simulink model "SmithVSPI"  (R2024b)
settings: Solver=VariableStepAuto  StartTime=0.0  StopTime=50000  FixedStep=10  RelTol=1e-3
undefined symbols (not defined in the file): n, p1, p2, p3, Vi
libraries: slpidlib x2
settings Model: Creator=HP  LastModifiedBy=HP

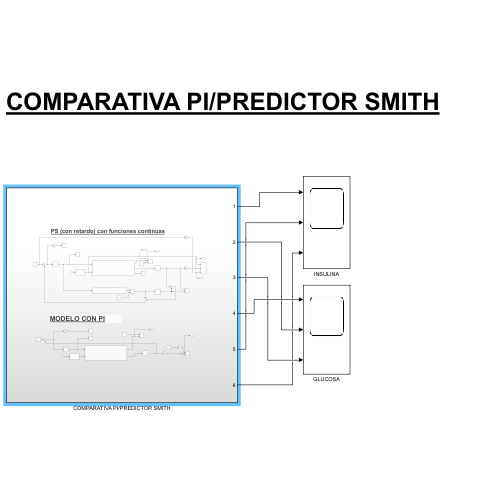
[thumbnail: Simulink's stored preview of the top-level diagram]
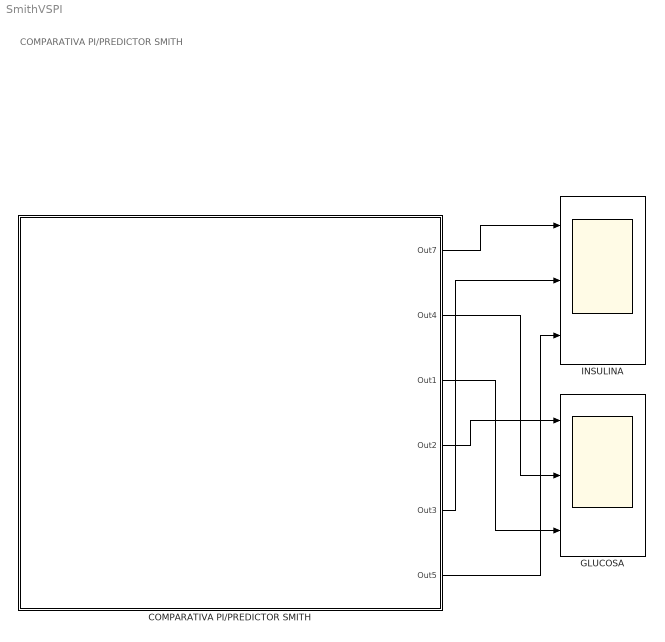
== system SmithVSPI ==
  note: COMPARATIVA PI/PREDICTOR SMITH
  COMPARATIVA PI/PREDICTOR SMITH : Subsystem
  GLUCOSA : Scope  NumInputPorts=3
  INSULINA : Scope  NumInputPorts=3
  wires:
  COMPARATIVA PI/PREDICTOR SMITH/2(Out4) -> GLUCOSA/2
  COMPARATIVA PI/PREDICTOR SMITH/3(Out1) -> GLUCOSA/3
  COMPARATIVA PI/PREDICTOR SMITH/4(Out2) -> GLUCOSA/1
  COMPARATIVA PI/PREDICTOR SMITH/1(Out7) -> INSULINA/1
  COMPARATIVA PI/PREDICTOR SMITH/5(Out3) -> INSULINA/2
  COMPARATIVA PI/PREDICTOR SMITH/6(Out5) -> INSULINA/3

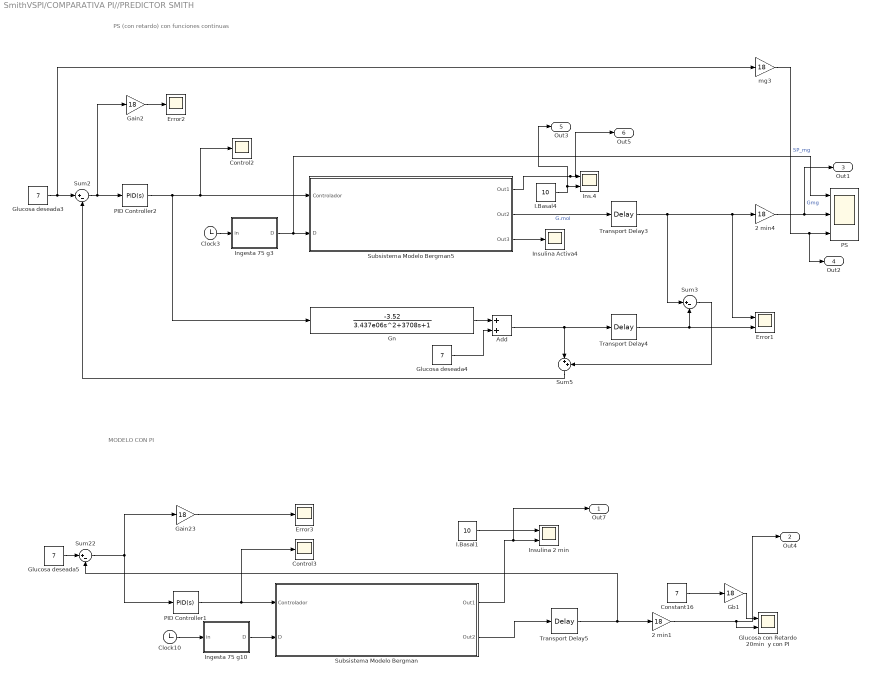
== system SmithVSPI/COMPARATIVA PI//PREDICTOR SMITH ==
  note: MODELO CON PI
  note: PS (con retardo) con funciones continuas
  2 min1 : Gain  Gain=18
  2 min4 : Gain  Gain=18
  Add : Sum
  Clock10 : Clock
  Clock3 : Clock
  Constant16 : Constant  Value=7
  Control2 : Scope
  Control3 : Scope
  Error1 : Scope  NumInputPorts=2
  Error2 : Scope
  Error3 : Scope
  Gain2 : Gain  Gain=18
  Gain23 : Gain  Gain=18
  Gb1 : Gain  Gain=18
  Glucosa con Retardo 20min  y con PI : Scope  NumInputPorts=2
  Glucosa deseada3 : Constant  Value=7
  Glucosa deseada4 : Constant  Value=7
  Glucosa deseada5 : Constant  Value=7
  Gn : TransferFcn  Numerator=[-3.52]  Denominator=[3.437e06 3708 1]
  I.Basal1 : Constant  Value=10
  I.Basal4 : Constant  Value=10
  Ingesta 75 g10 : MATLAB Function  TreatAsAtomicUnit=on
  Ingesta 75 g3 : MATLAB Function  TreatAsAtomicUnit=on
  Ins.4 : Scope  NumInputPorts=2
  Insulina 2 min : Scope  NumInputPorts=2
  Insulina Activa4 : Scope
  PID Controller1 : slpidlib/PID Controller  Controller=PID  Form=Parallel  TimeDomain=Continuous-time  UseExternalTs=off  SampleTime=-1  IntegratorMethod=Forward Euler  FilterMethod=Forward Euler  ControllerParametersSource=internal  P=-0.3195*1.5  I=-0.3195/2998.95  UseKiTs=off  D=0  UseExternalDerivativeSource=off  N=10  UseFilter=on  TunerSelectOption=Transfer Function Based (PID Tuner App)  InitialConditionSource=internal  InitialConditionForIntegrator=0  InitialConditionForFilter=0  DifferentiatorICPrevScaledInput=0  ExternalReset=none  TrackingMode=off  Kt=1  LimitOutput=on  SatLimitsSource=internal  UpperSaturationLimit=5  LowerSaturationLimit=0  LinearizeAsGain=on  AntiWindupMode=none  Kb=1  LimitIntegrator=off  UpperIntegratorSaturationLimit=inf  LowerIntegratorSaturationLimit=-inf  POutMin=[]  POutMax=[]  IOutMin=[]  IOutMax=[]  DOutMin=[]  DOutMax=[]  NOutMin=[]  NOutMax=[]  SumOutMin=[]  SumOutMax=[]  SaturationOutMin=[]  SaturationOutMax=[]  PParamMin=[]  PParamMax=[]  IParamMin=[]  IParamMax=[]  DParamMin=[]  DParamMax=[]  NParamMin=[]  NParamMax=[]  KbParamMin=[]  KbParamMax=[]  KtParamMin=[]  KtParamMax=[]  KbOutMin=[]  KbOutMax=[]  KtOutMin=[]  KtOutMax=[]  IntegratorOutMin=[]  IntegratorOutMax=[]  FilterOutMin=[]  FilterOutMax=[]  SumI1OutMin=[]  SumI1OutMax=[]  SumI2OutMin=[]  SumI2OutMax=[]  SumI3OutMin=[]  SumI3OutMax=[]  SumI4OutMin=[]  SumI4OutMax=[]  SumDOutMin=[]  SumDOutMax=[]  DifferentiatorOutMin=[]  DifferentiatorOutMax=[]  FilterDiffOutCoefMin=[]  FilterDiffOutCoefMax=[]  ReciprocalOutMin=[]  ReciprocalOutMax=[]  SumDenOutMin=[]  SumDenOutMax=[]  SumNumOutMin=[]  SumNumOutMax=[]  DivideOutMin=[]  DivideOutMax=[]  UdiffTsProdOutMin=[]  UdiffTsProdOutMax=[]  NTsProdOutMin=[]  NTsProdOutMax=[]  UintegralTsProdOutMin=[]  UintegralTsProdOutMax=[]  UngainTsProdOutMin=[]  UngainTsProdOutMax=[]  ClampingZeroOutDataTypeStr=Inherit: Inherit via back propagation  ClampingZeroOutMin=[]  ClampingZeroOutMax=[]  FilterDenConstantOutDataTypeStr=Inherit: Inherit via back propagation  FilterDenConstantOutMin=[]  FilterDenConstantOutMax=[]  PCopyOutDataTypeStr=Inherit: Inherit via back propagation  PCopyOutMin=[]  PCopyOutMax=[]  NCopyOutDataTypeStr=Inherit: Inherit via back propagation  NCopyOutMin=[]  NCopyOutMax=[]  IntegratorContinuousStateAttributes=''  IntegratorStateMustResolveToSignalObject=off  IntegratorRTWStateStorageClass=Auto  FilterContinuousStateAttributes=''  FilterStateMustResolveToSignalObject=off  FilterRTWStateStorageClass=Auto  ParallelPVariant=InternalParameters  IdealPVariant=Disabled  IVariant=InternalParameters  DVariant=InternalParameters  IntegratorVariant=Continuous  SatVariant=Enabled  AWVariant=Passthrough  PCopyVariant=Disabled  TRVariant=Disabled  FdbkBlocksVariant=Forward  IdealPFdbkVariant=Disabled  SatFdbkVariant=Disabled  DerivativeFilterVariant=ContFilter  NVariant=InternalParameters  NCopyVariant=Disabled  FilterICVariant=InternalICsFilter  IntegratorICVariant=InternalICs  ExternalResetVariant=Disabled  TRSumVariant=Passthrough  SumFdbkVariant=Disabled  SumVariant=Sum_PID  TsampFilterVariant=InternalTs  TsampNgainVariant=Passthrough  TsampIntegralVariant=Disabled_SignalSpec  ExternalSaturationOutDataTypeStr=Inherit: Same as second input  DerivativeSourceVariant=ErrorSignal  PreIntVariant=InternalPreInt
  PID Controller2 : slpidlib/PID Controller  Controller=PID  Form=Parallel  TimeDomain=Continuous-time  UseExternalTs=off  SampleTime=-1  IntegratorMethod=Forward Euler  FilterMethod=Forward Euler  ControllerParametersSource=internal  P=-0.3195*1.5  I=-0.3195/2998.95  UseKiTs=off  D=0  UseExternalDerivativeSource=off  N=10  UseFilter=on  TunerSelectOption=Transfer Function Based (PID Tuner App)  InitialConditionSource=internal  InitialConditionForIntegrator=0  InitialConditionForFilter=0  DifferentiatorICPrevScaledInput=0  ExternalReset=none  TrackingMode=off  Kt=1  LimitOutput=on  SatLimitsSource=internal  UpperSaturationLimit=5  LowerSaturationLimit=0  LinearizeAsGain=on  AntiWindupMode=none  Kb=1  LimitIntegrator=off  UpperIntegratorSaturationLimit=inf  LowerIntegratorSaturationLimit=-inf  POutMin=[]  POutMax=[]  IOutMin=[]  IOutMax=[]  DOutMin=[]  DOutMax=[]  NOutMin=[]  NOutMax=[]  SumOutMin=[]  SumOutMax=[]  SaturationOutMin=[]  SaturationOutMax=[]  PParamMin=[]  PParamMax=[]  IParamMin=[]  IParamMax=[]  DParamMin=[]  DParamMax=[]  NParamMin=[]  NParamMax=[]  KbParamMin=[]  KbParamMax=[]  KtParamMin=[]  KtParamMax=[]  KbOutMin=[]  KbOutMax=[]  KtOutMin=[]  KtOutMax=[]  IntegratorOutMin=[]  IntegratorOutMax=[]  FilterOutMin=[]  FilterOutMax=[]  SumI1OutMin=[]  SumI1OutMax=[]  SumI2OutMin=[]  SumI2OutMax=[]  SumI3OutMin=[]  SumI3OutMax=[]  SumI4OutMin=[]  SumI4OutMax=[]  SumDOutMin=[]  SumDOutMax=[]  DifferentiatorOutMin=[]  DifferentiatorOutMax=[]  FilterDiffOutCoefMin=[]  FilterDiffOutCoefMax=[]  ReciprocalOutMin=[]  ReciprocalOutMax=[]  SumDenOutMin=[]  SumDenOutMax=[]  SumNumOutMin=[]  SumNumOutMax=[]  DivideOutMin=[]  DivideOutMax=[]  UdiffTsProdOutMin=[]  UdiffTsProdOutMax=[]  NTsProdOutMin=[]  NTsProdOutMax=[]  UintegralTsProdOutMin=[]  UintegralTsProdOutMax=[]  UngainTsProdOutMin=[]  UngainTsProdOutMax=[]  ClampingZeroOutDataTypeStr=Inherit: Inherit via back propagation  ClampingZeroOutMin=[]  ClampingZeroOutMax=[]  FilterDenConstantOutDataTypeStr=Inherit: Inherit via back propagation  FilterDenConstantOutMin=[]  FilterDenConstantOutMax=[]  PCopyOutDataTypeStr=Inherit: Inherit via back propagation  PCopyOutMin=[]  PCopyOutMax=[]  NCopyOutDataTypeStr=Inherit: Inherit via back propagation  NCopyOutMin=[]  NCopyOutMax=[]  IntegratorContinuousStateAttributes=''  IntegratorStateMustResolveToSignalObject=off  IntegratorRTWStateStorageClass=Auto  FilterContinuousStateAttributes=''  FilterStateMustResolveToSignalObject=off  FilterRTWStateStorageClass=Auto  ParallelPVariant=InternalParameters  IdealPVariant=Disabled  IVariant=InternalParameters  DVariant=InternalParameters  IntegratorVariant=Continuous  SatVariant=Enabled  AWVariant=Passthrough  PCopyVariant=Disabled  TRVariant=Disabled  FdbkBlocksVariant=Forward  IdealPFdbkVariant=Disabled  SatFdbkVariant=Disabled  DerivativeFilterVariant=ContFilter  NVariant=InternalParameters  NCopyVariant=Disabled  FilterICVariant=InternalICsFilter  IntegratorICVariant=InternalICs  ExternalResetVariant=Disabled  TRSumVariant=Passthrough  SumFdbkVariant=Disabled  SumVariant=Sum_PID  TsampFilterVariant=InternalTs  TsampNgainVariant=Passthrough  TsampIntegralVariant=Disabled_SignalSpec  ExternalSaturationOutDataTypeStr=Inherit: Same as second input  DerivativeSourceVariant=ErrorSignal  PreIntVariant=InternalPreInt
  PS : Scope  NumInputPorts=3
  Subsistema Modelo Bergman : Subsystem
  Subsistema Modelo Bergman5 : Subsystem
  Sum2 : Sum  Inputs=|+-
  Sum22 : Sum  Inputs=|+-
  Sum3 : Sum  Inputs=|+-
  Sum5 : Sum  Inputs=|++
  Transport Delay3 : TransportDelay  DelayTime=900  InitialOutput=7
  Transport Delay4 : TransportDelay  DelayTime=900  InitialOutput=7
  Transport Delay5 : TransportDelay  DelayTime=1200  InitialOutput=7
  mg3 : Gain  Gain=18
  Out7 : Outport
  Out4 : Outport  Port=2
  Out1 : Outport  Port=3
  Out2 : Outport  Port=4
  Out3 : Outport  Port=5
  Out5 : Outport  Port=6
  wires:
  PID Controller1/1 -> Control3/1, Subsistema Modelo Bergman/1(Controlador)
  Subsistema Modelo Bergman/1(Out1) -> Out7/1, Insulina 2 min/2
  Glucosa deseada5/1 -> Sum22/1
  Subsistema Modelo Bergman/2(Out2) -> Transport Delay5/1
  Sum22/1 -> PID Controller1/1, Gain23/1
  Transport Delay5/1 -> Sum22/2, 2 min1/1
  Gb1/1 -> Glucosa con Retardo 20min  y con PI/1
  Ingesta 75 g10/1(D) -> Subsistema Modelo Bergman/2(D)
  I.Basal1/1 -> Insulina 2 min/1
  Gain23/1 -> Error3/1
  Clock10/1 -> Ingesta 75 g10/1(in)
  2 min1/1 -> Out4/1, Glucosa con Retardo 20min  y con PI/2
  Constant16/1 -> Gb1/1
  2 min4/1 -> Out1/1, PS/2  "Gmg"
  Add/1 -> Transport Delay4/1, Sum5/1
  Sum3/1 -> Sum5/2
  I.Basal4/1 -> Out3/1, Ins.4/2
  Gain2/1 -> Error2/1
  PID Controller2/1 -> Gn/1, Control2/1, Subsistema Modelo Bergman5/1(Controlador)
  Subsistema Modelo Bergman5/2(Out2) -> Transport Delay3/1  "G.mol"
  Subsistema Modelo Bergman5/3(Out3) -> Insulina Activa4/1
  Ingesta 75 g3/1(D) -> PS/1, Subsistema Modelo Bergman5/2(D)
  Gn/1 -> Add/1
  Subsistema Modelo Bergman5/1(Out1) -> Out5/1, Ins.4/1
  Sum5/1 -> Sum2/2
  Glucosa deseada4/1 -> Add/2
  mg3/1 -> Out2/1, PS/3  "SP_mg"
  Glucosa deseada3/1 -> mg3/1, Sum2/1
  Transport Delay3/1 -> Sum3/1, Error1/1, 2 min4/1
  Sum2/1 -> Gain2/1, PID Controller2/1
  Clock3/1 -> Ingesta 75 g3/1(in)
  Transport Delay4/1 -> Sum3/2, Error1/2

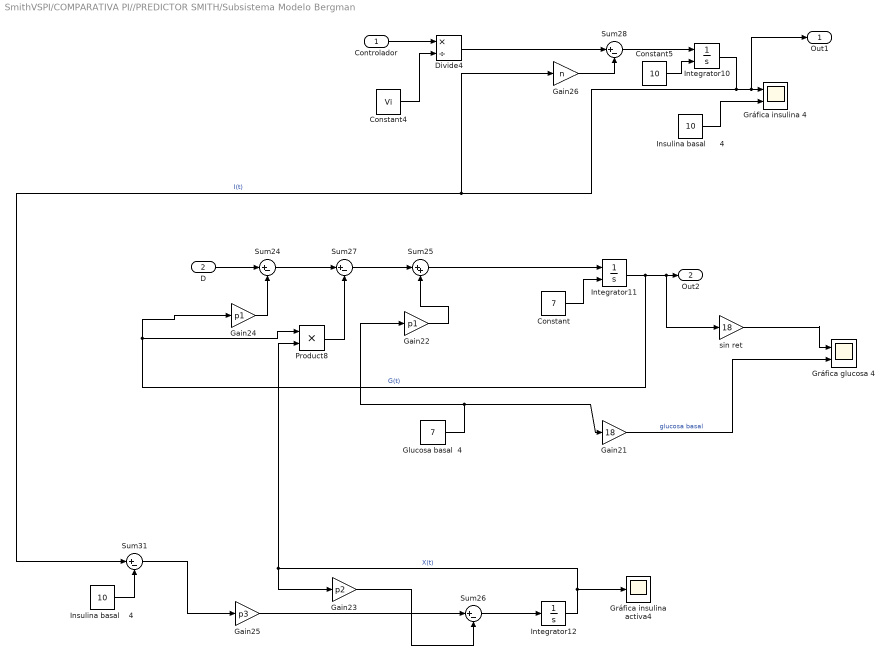
== system SmithVSPI/COMPARATIVA PI//PREDICTOR SMITH/Subsistema Modelo Bergman ==
  Controlador : Inport
  D : Inport  Port=2
  Constant : Constant  Value=7
  Constant4 : Constant  Value=Vi
  Constant5 : Constant  Value=10
  Divide4 : Product  Inputs=*/
  Gain21 : Gain  Gain=18
  Gain22 : Gain  Gain=p1
  Gain23 : Gain  Gain=p2
  Gain24 : Gain  Gain=p1
  Gain25 : Gain  Gain=p3
  Gain26 : Gain  Gain=n
  Glucosa basal  4 : Constant  Value=7
  Gráfica glucosa 4 : Scope  NumInputPorts=2
  Gráfica insulina 4 : Scope  NumInputPorts=2
  Gráfica insulina activa4 : Scope
  Insulina basal      4 : Constant  Value=10
  Insulina basal    4 : Constant  Value=10
  Integrator10 : Integrator  InitialConditionSource=external
  Integrator11 : Integrator  InitialConditionSource=external  InitialCondition=7
  Integrator12 : Integrator
  Product8 : Product
  Sum{24,26..28,31} (5 alike) : Sum  Inputs=|+-
  Sum25 : Sum  Inputs=|++
  sin ret : Gain  Gain=18
  Out1 : Outport
  Out2 : Outport  Port=2
  wires:
  Gain26/1 -> Sum28/2
  Glucosa basal  4/1 -> Gain22/1, Gain21/1
  D/1 -> Sum24/1
  Gain21/1 -> Gráfica glucosa 4/2  "glucosa basal"
  Integrator11/1 -> sin ret/1, Out2/1, Gain24/1, Product8/1  "G(t)"
  Integrator12/1 -> Product8/2, Gain23/1, Gráfica insulina activa4/1  "X(t)"
  Gain25/1 -> Sum26/1
  Integrator10/1 -> Out1/1, Gráfica insulina 4/1, Sum31/1, Gain26/1  "I(t)"
  Constant5/1 -> Integrator10/2
  Sum31/1 -> Gain25/1
  Sum26/1 -> Integrator12/1
  Gain23/1 -> Sum26/2
  Sum28/1 -> Integrator10/1
  Sum24/1 -> Sum27/1
  Sum25/1 -> Integrator11/1
  Gain24/1 -> Sum24/2
  Insulina basal      4/1 -> Gráfica insulina 4/2
  Sum27/1 -> Sum25/1
  Insulina basal    4/1 -> Sum31/2
  Divide4/1 -> Sum28/1
  Gain22/1 -> Sum25/2
  Product8/1 -> Sum27/2
  Constant4/1 -> Divide4/2
  Constant/1 -> Integrator11/2
  Controlador/1 -> Divide4/1
  sin ret/1 -> Gráfica glucosa 4/1

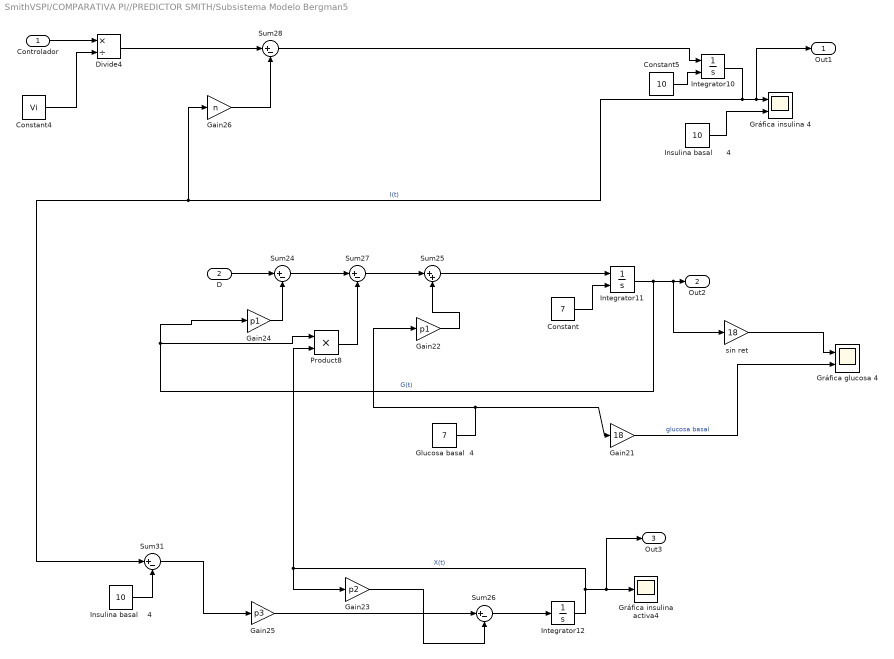
== system SmithVSPI/COMPARATIVA PI//PREDICTOR SMITH/Subsistema Modelo Bergman5 ==
  Controlador : Inport
  D : Inport  Port=2
  Constant : Constant  Value=7
  Constant4 : Constant  Value=Vi
  Constant5 : Constant  Value=10
  Divide4 : Product  Inputs=*/
  Gain21 : Gain  Gain=18
  Gain22 : Gain  Gain=p1
  Gain23 : Gain  Gain=p2
  Gain24 : Gain  Gain=p1
  Gain25 : Gain  Gain=p3
  Gain26 : Gain  Gain=n
  Glucosa basal  4 : Constant  Value=7
  Gráfica glucosa 4 : Scope  NumInputPorts=2
  Gráfica insulina 4 : Scope  NumInputPorts=2
  Gráfica insulina activa4 : Scope
  Insulina basal      4 : Constant  Value=10
  Insulina basal    4 : Constant  Value=10
  Integrator10 : Integrator  InitialConditionSource=external
  Integrator11 : Integrator  InitialConditionSource=external  InitialCondition=7
  Integrator12 : Integrator
  Product8 : Product
  Sum{24,26..28,31} (5 alike) : Sum  Inputs=|+-
  Sum25 : Sum  Inputs=|++
  sin ret : Gain  Gain=18
  Out1 : Outport
  Out2 : Outport  Port=2
  Out3 : Outport  Port=3
  wires:
  Gain26/1 -> Sum28/2
  Glucosa basal  4/1 -> Gain22/1, Gain21/1
  D/1 -> Sum24/1
  Gain21/1 -> Gráfica glucosa 4/2  "glucosa basal"
  Integrator11/1 -> sin ret/1, Out2/1, Gain24/1, Product8/1  "G(t)"
  Integrator12/1 -> Product8/2, Gain23/1, Out3/1, Gráfica insulina activa4/1  "X(t)"
  Gain25/1 -> Sum26/1
  Integrator10/1 -> Out1/1, Gráfica insulina 4/1, Sum31/1, Gain26/1  "I(t)"
  Constant5/1 -> Integrator10/2
  Sum31/1 -> Gain25/1
  Sum26/1 -> Integrator12/1
  Gain23/1 -> Sum26/2
  Sum28/1 -> Integrator10/1
  Sum24/1 -> Sum27/1
  Sum25/1 -> Integrator11/1
  Gain24/1 -> Sum24/2
  Insulina basal      4/1 -> Gráfica insulina 4/2
  Sum27/1 -> Sum25/1
  Insulina basal    4/1 -> Sum31/2
  Divide4/1 -> Sum28/1
  Gain22/1 -> Sum25/2
  Product8/1 -> Sum27/2
  Constant4/1 -> Divide4/2
  Constant/1 -> Integrator11/2
  Controlador/1 -> Divide4/1
  sin ret/1 -> Gráfica glucosa 4/1

== matlab function SmithVSPI/COMPARATIVA PI//PREDICTOR SMITH/Ingesta 75 g10 ==
  data: in input; D output
function D = comida(in)
% Variables de entrada en la funcion
t = in(1) %- 8*60*60; % Ajuste para iniciar a las 8 de la mañana
 
% Parámetros del modelo
Ag = 0.8; % adimensional
Tmaxi = 55*60; % s
Vg = 13.79; % L
Tmaxg = 40*60; % s
t1 = 0;
Dg = 0;
f = 1000/180; % factor de conversión de g a mmol
 
% Comidas (perturbaciones) a lo largo de un día
Dg = 50*f;
 
% Ecuación
D = (Dg*Ag*(t-t1)*exp(-(t-t1)/Tmaxi))/(Vg*Tmaxg^2);

== matlab function SmithVSPI/COMPARATIVA PI//PREDICTOR SMITH/Ingesta 75 g3 ==
  data: in input; D output
function D = comida(in)
% Variables de entrada en la funcion
t = in(1) %- 8*60*60; % Ajuste para iniciar a las 8 de la mañana
 
% Parámetros del modelo
Ag = 0.8; % adimensional
Tmaxi = 55*60; % s
Vg = 13.79; % L
Tmaxg = 40*60; % s
t1 = 1000;
Dg = 0;
f = 1000/180; % factor de conversión de g a mmol
 
% Comidas (perturbaciones) a lo largo de un día
Dg = 50*f;
 
% Ecuación
if (t <= t1)
    D = 0;
else
    D = (Dg*Ag*(t-t1)*exp(-(t-t1)/Tmaxi))/(Vg*Tmaxg^2);
end
